simulink subsystem "motor_drive"  (R2022b)
settings: Solver=VariableStepAuto  StartTime=0.0  StopTime=10.0  RelTol=1e-3
model mask{pwm_pin=D9, dir_pin=D5, flip_direction=off}
  mask prompts: pwm_pin "PWM Pin"; dir_pin "Direction Pin"; flip_direction "Flip Direction"
libraries: mbedblockslib x2, simulink x1
settings Model: Creator=micha  LastModifiedBy=micha

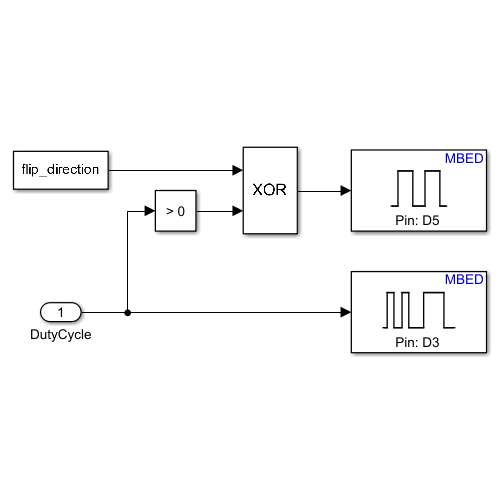
[thumbnail: Simulink's stored preview of the top-level diagram]
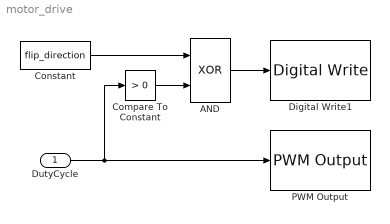
== system motor_drive ==
  DutyCycle : Inport
  AND : Logic  Operator=XOR  AllPortsSameDT=off  OutDataTypeStr=boolean
  Compare To Constant : simulink/Logic and Bit Operations/Compare To Constant  relop=>  const=0  OutDataTypeStr=boolean
  Constant : Constant  Value=flip_direction  OutDataTypeStr=boolean
  Digital Write1 : mbedblockslib/Digital Write  Pin=D2  Direction=output
      settings: LibrarySourceBlock=stmnucleorootlib/Common/Digital Write
  PWM Output : mbedblockslib/PWM Output  Pin=D9  EnableInputFrequency=off  InitialFrequency=2000  InitialDutyCycle=0  NotificationType=None
      settings: LibrarySourceBlock=stmnucleorootlib/Common/PWM Output
  wires:
  DutyCycle/1 -> Compare To Constant/1, PWM Output/1
  Compare To Constant/1 -> AND/2
  Constant/1 -> AND/1
  AND/1 -> Digital Write1/1
